simulink model "motor_kit_sim_20MHz"  (R2021b)
settings: Solver=VariableStepAuto  StartTime=0.0  StopTime=10*62.5E-6  RelTol=1e-3  EnableMultiTasking=on
PreLoadFcn:
  | setup_motor_kit_sim_20MHz;
InitFcn:
  | setup_motor_kit_sim_20MHz;
values from neighbouring files (symbols this model uses):
  DSPBASampleTime = 0.05e-6    (= 5e-08)    [setup_motor_kit_sim_20MHz.m]
  wordLength = 16    [setup_motor_kit_sim_20MHz.m]
undefined symbols (not defined in the file or in its folder): AdvDSPBChannelOutDisplay, dpoly, dspba_ChannelInVis, dspba_ChannelOutVis, dspba_internal_get_channel_ports, evalAionMaskParam, latency, primtype, value, x
libraries: DSPBAPrim x324, DSPBAModelBus x25, DSPBABase x7, dspsrcs4 x3, simulink x3, DSPBAUtilities x1
(part 1 of 5)
settings Model: Creator=ksmith  LastModifiedBy=alexhunt
settings SolverCC: AlgebraicLoopSolver=TrustRegion
settings DataIOCC: LimitDataPoints=on  SaveFormat=StructureWithTime  SignalLoggingSaveFormat=ModelDataLogs  ReturnWorkspaceOutputs=off
settings OptimizationCC: ExpressionDepthLimit=2147483647  LifeSpan=inf
settings DebuggingCC: UnderspecifiedInitializationDetection=Classic  MergeDetectMultiDrivingBlocksExec=none  SolverPrmCheckMsg=warning  FcnCallInpInsideContextMsg=warning  StateNameClashWarn=warning  SFUnexpectedBacktrackingDiag=warning  SFNoUnconditionalDefaultTransitionDiag=warning  SFExecutionAtInitializationDiag=none  SFMachineParentedDataDiag=warning  ArithmeticOperatorsInVariantConditions=warning
settings HardwareCC: ProdBitPerPointer=32  ProdBitPerSizeT=32  ProdBitPerPtrDiffT=32  ProdLargestAtomicFloat=None  ProdIntDivRoundTo=Undefined  ProdEndianess=Unspecified  ProdWordSize=32  ProdHWDeviceType=32-bit Generic
settings ModelReferenceCC: PropagateSignalLabelsOutOfModel=off
settings SFSimCC: SimUseLocalCustomCode=off  CustomCodeUndefinedFunction=UseInterfaceOnly
settings RTWCC: RTWUseLocalCustomCode=off
settings CodeAppCC: StateflowObjectComments=on
settings GRTTargetCC: TargetLangStandard=C89/C90 (ANSI)  CombineOutputUpdateFcns=off  GRTInterface=on
settings ConfigComp: CovMetricSettings=dw  CovSaveCumulativeToWorkspaceVar=on  CovSaveSingleToWorkspaceVar=on  CovExternalEMLEnable=off

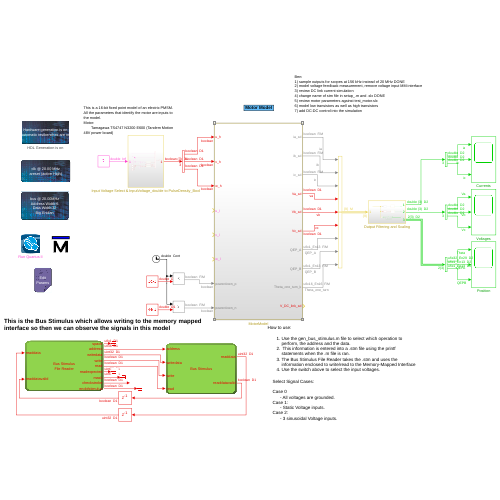
[thumbnail: Simulink's stored preview of the top-level diagram]
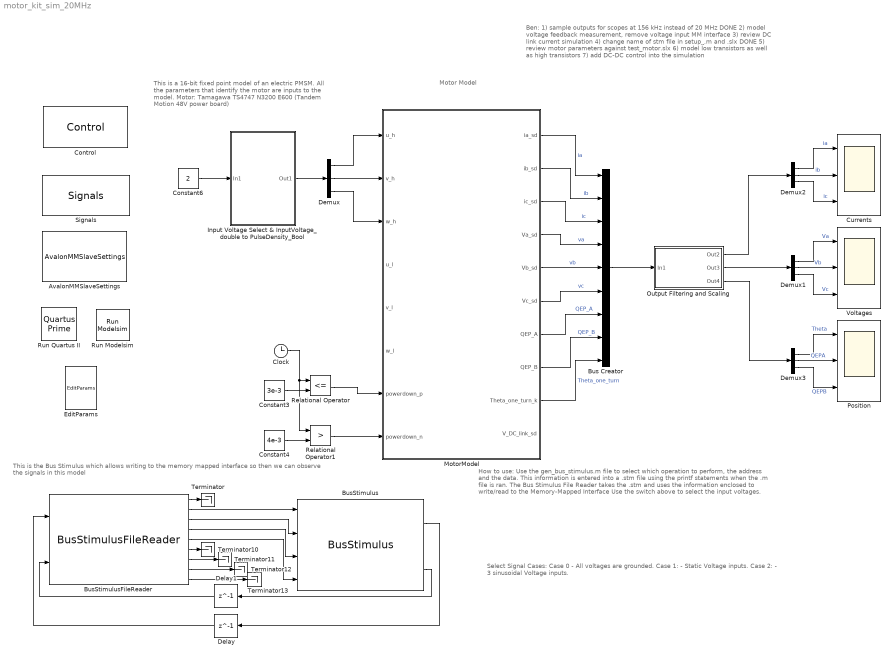
== system motor_kit_sim_20MHz ==
  note: Ben:
      | 1) sample outputs for scopes at 156 kHz instead of 20 MHz DONE
      | 2) model voltage feedback measurement, remove voltage input MM interface
      | 3) review DC link current simulation
      | 4) change name of stm file in setup_.m and .slx DONE
      | 5) review motor parameters against test_motor.slx
      | 6) model low transistors as well as high transistors
      | 7) add DC-DC control into the simulation
  note: How to use:
      |
      | Use the gen_bus_stimulus.m file to select which operation to perform, the address and the data.
      | This information is entered into a .stm file using the printf statements when the .m file is ran.
      | The Bus Stimulus File Reader takes the .stm and uses the information enclosed to write/read to the Memory-Mapped Interface
      | Use the switch above to select the input voltages.
  note: This is the Bus Stimulus which allows writing to the memory mapped interface so then we can observe the signals in this model
  note: This is a 16-bit fixed point model of an electric PMSM.
      | All the parameters that identify the motor are inputs to the model.
      | Motor:
      | 	Tamagawa TS4747 N3200 E600 (Tandem Motion 48V power board)
  note: Motor Model
  note: Select Signal Cases:
      |
      | Case 0
      | - All voltages are grounded.
      | Case 1:
      | - Static Voltage inputs.
      | Case 2:
      | - 3 sinusoidal Voltage inputs.
  AvalonMMSlaveSettings : DSPBABase/AvalonMMSlaveSettings
  Bus Creator : BusCreator  Inputs=9
  BusStimulus : DSPBAModelBus/BusStimulus  SampleTime=DSPBASampleTime  version=20140122  hasreaden=on
  BusStimulusFileReader : DSPBAModelBus/BusStimulusFileReader  enabled=on  filename=.\motor_kit_sim_20MHz_Autogen.stm  logfilename=.\test_bus_stimulus.bus.log  spacewidth=1  addrwidth=6  datawidth=32  SampleTime=DSPBASampleTime  version=20140124  hasreaden=on
  Clock : Clock
  Constant3 : Constant  Value=3e-3  OutDataTypeStr=double  SampleTime=DSPBASampleTime
  Constant4 : Constant  Value=4e-3  OutDataTypeStr=double  SampleTime=DSPBASampleTime
  Constant6 : Constant  Value=2
  Control : DSPBABase/Control  generate=on  language=VHDL  destination=./rtlmax10  destination_gui=./rtlmax10  make_full_path=off  path_is_relative=on  autotestbench=on  signaldepth=2  coveragetestbench=off  logs=off  spacewidth=2  spacenum=1  addrwidth=6  datawidth=32  dataendian=Big Endian  hierarchicalnames=off  ramThresholdBits=-1  distRamThresholdBits=-1  mlabThresholdBits=-1  hardMultiplierThresholdLuts=-1  version=20090407  errorOnChanMismatch=1  errorOnGPIOMismatch=0  importModelsimResults=0  cycleAccurate=off  reinterpretCastMult=off  paramFile=motor_kit_sim_20MHz_params.xml
      settings: AttributesFormatString=HDL Generation is %<generate>
  Currents : Scope  NumInputPorts=3
  Delay : Delay  DelayLength=1  InitialCondition=0
  Delay1 : Delay  DelayLength=1  InitialCondition=0
  Demux{,1..3} (4 alike) : Demux  Outputs=3
  EditParams : DSPBABase/EditParams  version=20090407
  Input Voltage Select & InputVoltage_double to PulseDensity_Bool : Subsystem
  MotorModel : Subsystem
  Output Filtering and Scaling : Subsystem
  Position : Scope  NumInputPorts=3
  Relational Operator : RelationalOperator  Operator=<=  OutDataTypeStr=boolean  RndMeth=Simplest
  Relational Operator1 : RelationalOperator  Operator=>  OutDataTypeStr=boolean  RndMeth=Simplest
  Run Modelsim : DSPBABase/Run Modelsim  version=20090407
  Run Quartus II : DSPBABase/Quartus Prime  version=20090407
  Signals : DSPBABase/Signals  clk=clk  freq=ClockFrequency  margin=0  rst=areset  rstactive=High  bus=bus  enbusclock=off  busfreq=20  bussync=on  version=20090407
  Terminator{,10..13} (5 alike) : Terminator
  Voltages : Scope  NumInputPorts=3
  wires:
  BusStimulusFileReader/2 -> BusStimulus/1
  BusStimulusFileReader/3 -> BusStimulus/2
  BusStimulusFileReader/4 -> BusStimulus/3
  BusStimulusFileReader/1 -> Terminator/1
  BusStimulusFileReader/6 -> Terminator10/1
  BusStimulusFileReader/7 -> Terminator11/1
  BusStimulusFileReader/8 -> Terminator12/1
  BusStimulusFileReader/9 -> Terminator13/1
  Delay/1 -> BusStimulusFileReader/1
  Delay1/1 -> BusStimulusFileReader/2
  BusStimulus/2 -> Delay1/1
  BusStimulus/1 -> Delay/1
  Demux/1 -> MotorModel/1(u_h)
  Demux/2 -> MotorModel/2(v_h)
  Demux/3 -> MotorModel/3(w_h)
  Demux1/1 -> Voltages/1  "Va"
  Demux1/2 -> Voltages/2  "Vb"
  Demux1/3 -> Voltages/3  "Vc"
  Demux2/1 -> Currents/1  "ia"
  Demux2/2 -> Currents/2  "ib"
  Demux2/3 -> Currents/3  "ic"
  Constant6/1 -> Input Voltage Select & InputVoltage_double to PulseDensity_Bool/1(In1)
  MotorModel/1(ia_sd) -> Bus Creator/1  "ia"
  MotorModel/2(ib_sd) -> Bus Creator/2  "ib"
  MotorModel/3(ic_sd) -> Bus Creator/3  "ic"
  MotorModel/4(Va_sd) -> Bus Creator/4  "va"
  MotorModel/5(Vb_sd) -> Bus Creator/5  "vb"
  MotorModel/6(Vc_sd) -> Bus Creator/6  "vc"
  MotorModel/7(QEP_A) -> Bus Creator/7  "QEP_A"
  MotorModel/8(QEP_B) -> Bus Creator/8  "QEP_B"
  MotorModel/9(Theta_one_turn_k) -> Bus Creator/9  "Theta_one_turn"
  Bus Creator/1 -> Output Filtering and Scaling/1(In1)
  Demux3/1 -> Position/1  "Theta"
  Demux3/2 -> Position/2  "QEPA"
  Demux3/3 -> Position/3  "QEPB"
  Output Filtering and Scaling/1(Out2) -> Demux2/1
  Output Filtering and Scaling/2(Out3) -> Demux1/1
  Output Filtering and Scaling/3(Out4) -> Demux3/1
  Input Voltage Select & InputVoltage_double to PulseDensity_Bool/1(Out1) -> Demux/1
  BusStimulusFileReader/5 -> BusStimulus/4
  Clock/1 -> Relational Operator1/1, Relational Operator/1
  Constant3/1 -> Relational Operator/2
  Constant4/1 -> Relational Operator1/2
  Relational Operator/1 -> MotorModel/7(powerdown_p)
  Relational Operator1/1 -> MotorModel/8(powerdown_n)

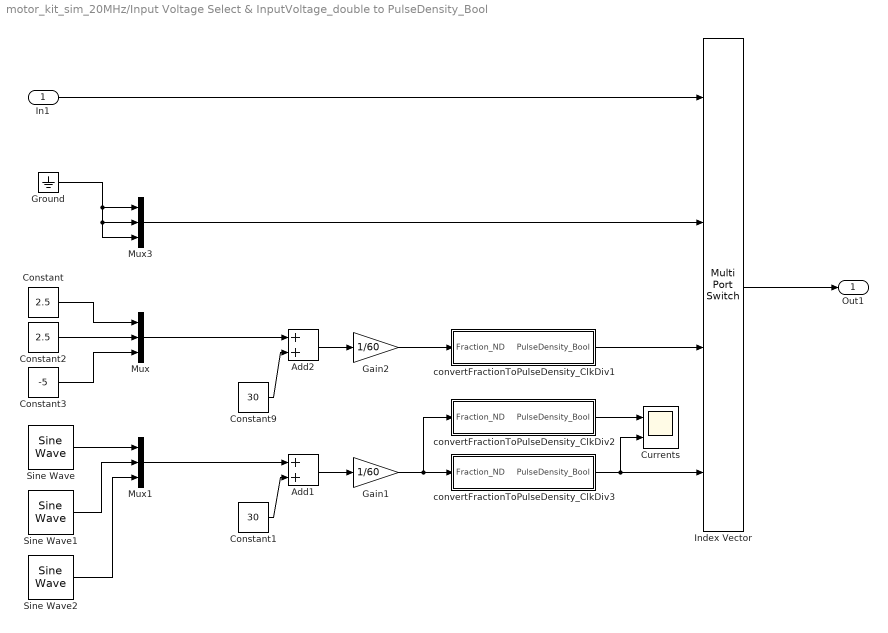
== system motor_kit_sim_20MHz/Input Voltage Select & InputVoltage_double to PulseDensity_Bool ==
  In1 : Inport
  Add1 : Sum
  Add2 : Sum
  Constant : Constant  Value=2.5
  Constant1 : Constant  Value=30
  Constant2 : Constant  Value=2.5
  Constant3 : Constant  Value=-5
  Constant9 : Constant  Value=30
  Currents : Scope  NumInputPorts=2
  Gain1 : Gain  Gain=1/60
  Gain2 : Gain  Gain=1/60
  Ground : Ground
  Index Vector : MultiPortSwitch  DataPortOrder=Zero-based contiguous  zeroidx=on
  Mux : Mux  Inputs=3
  Mux1 : Mux  Inputs=3
  Mux3 : Mux  Inputs=3
  Sine Wave : dspsrcs4/Sine Wave  Amplitude=2  Frequency=16.6  Phase=0  SampleMode=Discrete  OutComplex=Real  CompMethod=Trigonometric fcn  TableSize=Speed  SampleTime=1/20000000  SamplesPerFrame=1  ResetState=Restart at time zero  OutputFrames=off  dataType=double  wordLen=16  udDataType=sfix(16)  fracBitsMode=Best precision  numFracBits=15  OutDataTypeStr=double  LastOutDataTypeStr=double
  Sine Wave1 : dspsrcs4/Sine Wave  Amplitude=2  Frequency=16.6  Phase=2.094  SampleMode=Discrete  OutComplex=Real  CompMethod=Trigonometric fcn  TableSize=Speed  SampleTime=1/20000000  SamplesPerFrame=1  ResetState=Restart at time zero  OutputFrames=off  dataType=double  wordLen=16  udDataType=sfix(16)  fracBitsMode=Best precision  numFracBits=15  OutDataTypeStr=double  LastOutDataTypeStr=double
  Sine Wave2 : dspsrcs4/Sine Wave  Amplitude=2  Frequency=16.6  Phase=4.189  SampleMode=Discrete  OutComplex=Real  CompMethod=Trigonometric fcn  TableSize=Speed  SampleTime=1/20000000  SamplesPerFrame=1  ResetState=Restart at time zero  OutputFrames=off  dataType=double  wordLen=16  udDataType=sfix(16)  fracBitsMode=Best precision  numFracBits=15  OutDataTypeStr=double  LastOutDataTypeStr=double
  convertFractionToPulseDensity_ClkDiv1 : Subsystem
  convertFractionToPulseDensity_ClkDiv2 : Subsystem
  convertFractionToPulseDensity_ClkDiv3 : Subsystem
  Out1 : Outport
  wires:
  Add2/1 -> Gain2/1
  Constant9/1 -> Add2/2
  Gain2/1 -> convertFractionToPulseDensity_ClkDiv1/1(Fraction_ND)
  Constant1/1 -> Add1/2
  Add1/1 -> Gain1/1
  Mux1/1 -> Add1/1
  Constant2/1 -> Mux/2
  Constant/1 -> Mux/1
  Mux/1 -> Add2/1
  Constant3/1 -> Mux/3
  Sine Wave/1 -> Mux1/1
  Sine Wave1/1 -> Mux1/2
  Sine Wave2/1 -> Mux1/3
  convertFractionToPulseDensity_ClkDiv1/1(PulseDensity_Bool) -> Index Vector/3
  In1/1 -> Index Vector/1
  Ground/1 -> Mux3/3, Mux3/2, Mux3/1
  Mux3/1 -> Index Vector/2
  Index Vector/1 -> Out1/1
  convertFractionToPulseDensity_ClkDiv3/1(PulseDensity_Bool) -> Currents/2, Index Vector/4
  Gain1/1 -> convertFractionToPulseDensity_ClkDiv2/1(Fraction_ND), convertFractionToPulseDensity_ClkDiv3/1(Fraction_ND)
  convertFractionToPulseDensity_ClkDiv2/1(PulseDensity_Bool) -> Currents/1

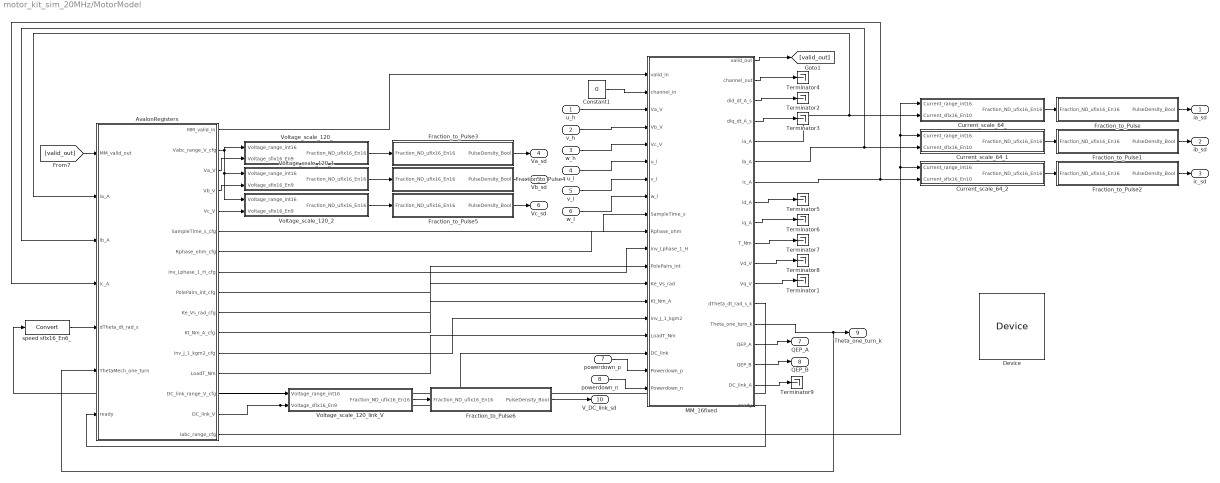
== system motor_kit_sim_20MHz/MotorModel ==
  u_h : Inport  OutDataTypeStr=boolean
  v_h : Inport  Port=2  OutDataTypeStr=boolean
  w_h : Inport  Port=3  OutDataTypeStr=boolean
  u_l : Inport  Port=4  OutDataTypeStr=boolean  PortDimensions=1
  v_l : Inport  Port=5  OutDataTypeStr=boolean  PortDimensions=1
  w_l : Inport  Port=6  OutDataTypeStr=boolean  PortDimensions=1
  powerdown_p : Inport  Port=7  OutDataTypeStr=boolean  PortDimensions=1
  powerdown_n : Inport  Port=8  OutDataTypeStr=boolean  PortDimensions=1
  AvalonRegisters : Subsystem
  Constant1 : Constant  Value=0  OutDataTypeStr=uint8
  Current_scale_64_ : Subsystem
  Current_scale_64_1 : Subsystem
  Current_scale_64_2 : Subsystem
  Device : DSPBABase/Device  family=MAX 10  deviceMember=Stratix V GX  stratix4device=Stratix IV E  hardcopy4device=HardCopy IV E  stratix5device=Stratix V GX  device=AUTO  speed=6  stratixSpeed=-5  stratix2Speed=-3  stratix3Speed=-2  stratix4gxSpeed=-2  stratix4gtSpeed=-1  cyclone2Speed=-6  cyclone3Speed=-7  arria2Speed=-4  cyclone4eSpeed=-8  stratix5Speed=-3  arria5Speed=-4  arriaSpeed=-6  cyclone3lsSpeed=-7  cyclone5Speed=-6  arria2gzSpeed=-3  nightFurySpeed=-2  ecp2Speed=-7  hardcopycompat=off  version=20140217  max10flashmode=off  max10nomeminit=off
  Fraction_to_Pulse : Subsystem
  Fraction_to_Pulse1 : Subsystem
  Fraction_to_Pulse2 : Subsystem
  Fraction_to_Pulse3 : Subsystem
  Fraction_to_Pulse4 : Subsystem
  Fraction_to_Pulse5 : Subsystem
  Fraction_to_Pulse6 : Subsystem
  MM_16fixed : Subsystem
  Terminator{1..9} (9 alike) : Terminator
  Voltage_scale_120_ : Subsystem
  Voltage_scale_120_1 : Subsystem
  Voltage_scale_120_2 : Subsystem
  Voltage_scale_120_link_V : Subsystem
  speed sfix16_En6_ : DSPBAPrim/Convert  primtype=convert  nInputs=1  nOutputs=1  omode=Specify via dialog  otype=sfix(16)  scale=2^-6  rndmethod=Unbiased  factor=1  satmethod=None  shift_vec=[0 1 2 -1]  value=round([0:255]/17)  inPortNames=[' '; ' ';]  outPortNames=[' '; 'c']  dspbaimage=dspba_prim_wide.svg  text=fprintf('convert');  style=Optimised  visibilities=8+64+256+2^17  clipdetect=off  floatPrecision=float32_m23  advOptions=[]  version=20211007
  ia_sd : Outport
  ib_sd : Outport  Port=2
  ic_sd : Outport  Port=3
  Va_sd : Outport  Port=4
  Vb_sd : Outport  Port=5
  Vc_sd : Outport  Port=6
  QEP_A : Outport  Port=7
  QEP_B : Outport  Port=8
  Theta_one_turn_k : Outport  Port=9
  V_DC_link_sd : Outport  Port=10
  wires:
  Fraction_to_Pulse4/1("PulseDensity_Bool ") -> Vb_sd/1
  Fraction_to_Pulse2/1("PulseDensity_Bool ") -> ic_sd/1
  MM_16fixed/6(ib_A) -> AvalonRegisters/3(ib_A), Current_scale_64_1/2(Current_sfix16_En10)
  MM_16fixed/7(ic_A) -> Current_scale_64_2/2(Current_sfix16_En10), AvalonRegisters/4(ic_A)
  MM_16fixed/12(Vq_V) -> Terminator1/1
  [valid_out] -> AvalonRegisters/1(MM_valid_out)
  MM_16fixed/9(iq_A) -> Terminator6/1
  MM_16fixed/13(dTheta_dt_rad_s_k) -> speed sfix16_En6_/1
  MM_16fixed/4(diq_dt_A_s) -> Terminator3/1
  MM_16fixed/3(did_dt_A_s) -> Terminator2/1
  MM_16fixed/10(T_Nm) -> Terminator7/1
  AvalonRegisters/9(PolePairs_int_cfg) -> MM_16fixed/12(PolePairs_int)
  AvalonRegisters/12(inv_J_1_kgm2_cfg) -> MM_16fixed/15(inv_J_1_kgm2)
  AvalonRegisters/1(MM_valid_in) -> MM_16fixed/1(valid_in)
  AvalonRegisters/10(Ke_Vs_rad_cfg) -> MM_16fixed/13(Ke_Vs_rad)
  AvalonRegisters/8(inv_Lphase_1_H_cfg) -> MM_16fixed/11(inv_Lphase_1_H)
  Fraction_to_Pulse5/1("PulseDensity_Bool ") -> Vc_sd/1
  AvalonRegisters/11(Kt_Nm_A_cfg) -> MM_16fixed/14(Kt_Nm_A)
  AvalonRegisters/7(Rphase_ohm_cfg) -> MM_16fixed/10(Rphase_ohm)
  Fraction_to_Pulse1/1("PulseDensity_Bool ") -> ib_sd/1
  MM_16fixed/5(ia_A) -> Current_scale_64_/2(Current_sfix16_En10), AvalonRegisters/2(ia_A)
  MM_16fixed/11(Vd_V) -> Terminator8/1
  MM_16fixed/2(channel_out) -> Terminator4/1
  AvalonRegisters/6(SampleTime_s_cfg) -> MM_16fixed/9(SampleTime_s)
  speed sfix16_En6_/1 -> AvalonRegisters/5(dTheta_dt_rad_s)
  MM_16fixed/8(id_A) -> Terminator5/1
  AvalonRegisters/13(LoadT_Nm) -> MM_16fixed/16(LoadT_Nm)
  MM_16fixed/18(ready) -> AvalonRegisters/7(ready)
  MM_16fixed/1(valid_out) -> [valid_out]
  Constant1/1 -> MM_16fixed/2(channel_in)
  MM_16fixed/15(QEP_A) -> QEP_A/1
  MM_16fixed/16(QEP_B) -> QEP_B/1
  MM_16fixed/14(Theta_one_turn_k) -> AvalonRegisters/6(ThetaMech_one_turn), Theta_one_turn_k/1
  v_h/1 -> MM_16fixed/4(Vb_V)
  w_h/1 -> MM_16fixed/5(Vc_V)
  Fraction_to_Pulse3/1("PulseDensity_Bool ") -> Va_sd/1
  Fraction_to_Pulse/1("PulseDensity_Bool ") -> ia_sd/1
  u_h/1 -> MM_16fixed/3(Va_V)
  Voltage_scale_120_/1("Fraction_ND_ufix16_En16 ") -> Fraction_to_Pulse3/1(Fraction_ND_ufix16_En16)
  Voltage_scale_120_2/1("Fraction_ND_ufix16_En16 ") -> Fraction_to_Pulse5/1(Fraction_ND_ufix16_En16)
  Voltage_scale_120_1/1("Fraction_ND_ufix16_En16 ") -> Fraction_to_Pulse4/1(Fraction_ND_ufix16_En16)
  Current_scale_64_1/1("Fraction_ND_ufix16_En16 ") -> Fraction_to_Pulse1/1(Fraction_ND_ufix16_En16)
  Current_scale_64_/1("Fraction_ND_ufix16_En16 ") -> Fraction_to_Pulse/1(Fraction_ND_ufix16_En16)
  Current_scale_64_2/1("Fraction_ND_ufix16_En16 ") -> Fraction_to_Pulse2/1(Fraction_ND_ufix16_En16)
  AvalonRegisters/15(DC_link_V) -> MM_16fixed/17(DC_link), Voltage_scale_120_link_V/2(Voltage_sfix16_En9)
  w_l/1 -> MM_16fixed/8(w_l)
  v_l/1 -> MM_16fixed/7(v_l)
  u_l/1 -> MM_16fixed/6(u_l)
  Voltage_scale_120_link_V/1("Fraction_ND_ufix16_En16 ") -> Fraction_to_Pulse6/1(Fraction_ND_ufix16_En16)
  Fraction_to_Pulse6/1("PulseDensity_Bool ") -> V_DC_link_sd/1
  MM_16fixed/17(DC_link_A) -> Terminator9/1
  AvalonRegisters/5(Vc_V) -> Voltage_scale_120_2/2(Voltage_sfix16_En9)
  AvalonRegisters/4(Vb_V) -> Voltage_scale_120_1/2(Voltage_sfix16_En9)
  AvalonRegisters/3(Va_V) -> Voltage_scale_120_/2(Voltage_sfix16_En9)
  AvalonRegisters/2(Vabc_range_V_cfg) -> Voltage_scale_120_2/1(Voltage_range_int16), Voltage_scale_120_1/1(Voltage_range_int16), Voltage_scale_120_/1(Voltage_range_int16)
  AvalonRegisters/14(DC_link_range_V_cfg) -> Voltage_scale_120_link_V/1(Voltage_range_int16)
  AvalonRegisters/16(Iabc_range_cfg) -> Current_scale_64_/1(Current_range_int16), Current_scale_64_1/1(Current_range_int16), Current_scale_64_2/1(Current_range_int16)
  powerdown_p/1 -> MM_16fixed/18(Powerdown_p)
  powerdown_n/1 -> MM_16fixed/19(Powerdown_n)

== system motor_kit_sim_20MHz/Output Filtering and Scaling ==
  In1 : Inport
  Bus Creator : BusCreator  Inputs=3
  Bus Selector : BusSelector  OutputSignals=ia,ib,ic  OutputAsBus=on
  Bus Selector1 : BusSelector  OutputSignals=va,vb,vc  OutputAsBus=on
  Bus Selector2 : BusSelector  OutputSignals=Theta_one_turn,QEP_A,QEP_B
  Data Type Conversion : DataTypeConversion  OutDataTypeStr=double
  Data Type Conversion1 : DataTypeConversion  OutDataTypeStr=double
  Gain3 : Gain  Gain=2*pi
  Sinc3 Filter : Subsystem
  Sinc3 Filter1 : Subsystem
  Zero-Order Hold : ZeroOrderHold  SampleTime=128*DSPBASampleTime
  Out2 : Outport
  Out3 : Outport  Port=2
  Out4 : Outport  Port=3
  wires:
  Bus Selector/1 -> Data Type Conversion/1
  Bus Selector1/1 -> Data Type Conversion1/1
  Bus Selector2/1 -> Gain3/1  "<Theta_one_turn>"
  Gain3/1 -> Bus Creator/1
  Bus Selector2/3 -> Bus Creator/3  "<QEP_B>"
  Bus Selector2/2 -> Bus Creator/2  "<QEP_A>"
  Bus Creator/1 -> Out4/1
  In1/1 -> Zero-Order Hold/1, Bus Selector1/1, Bus Selector/1
  Data Type Conversion1/1 -> Sinc3 Filter/1(In1)
  Data Type Conversion/1 -> Sinc3 Filter1/1(In1)
  Sinc3 Filter1/1(Out1) -> Out2/1
  Sinc3 Filter/1(Out1) -> Out3/1
  Zero-Order Hold/1 -> Bus Selector2/1

== system motor_kit_sim_20MHz/Input Voltage Select & InputVoltage_double to PulseDensity_Bool/convertFractionToPulseDensity_ClkDiv1 ==
  note: Subtract threshold once it is reached
  note: Each timestep:
      | Calculate the new value of the integral:
      | New value (temp) =  Old value + input*timestep
      | If the new value exceeds the threshold:
      | 1. Set output to 1
      | 2. Decrease the integral by the threshold:
      | New value (final) =  New value (temp) - threshold
      | Else
      | 1. Set output to zero
      | 2. New value (final) =  New value (temp)
  Fraction_ND : Inport
  Compare To Threshold : simulink/Logic and Bit Operations/Compare To Constant  relop=>=  const=1  OutDataTypeStr=boolean
  Constant : Constant
  Constant1 : Constant  Value=0
  Rate Transition : RateTransition  OutPortSampleTime=DSPBASampleTime
  Rate Transition1 : RateTransition  OutPortSampleTime=DSPBASampleTime
  Sum : Sum  Inputs=+-
  Sum1 : Sum
  Switch : Switch  Criteria=u2 > Threshold
  Unit Delay1 : UnitDelay  SampleTime=-1  HasFrameUpgradeWarning=on
  PulseDensity_Bool : Outport
  wires:
  Switch/1 -> Sum/2
  Constant1/1 -> Switch/3
  Constant/1 -> Switch/1
  Unit Delay1/1 -> Sum1/2, Compare To Threshold/1
  Sum1/1 -> Unit Delay1/1
  Compare To Threshold/1 -> Switch/2, Rate Transition/1
  Fraction_ND/1 -> Rate Transition1/1
  Sum/1 -> Sum1/1
  Rate Transition1/1 -> Sum/1
  Rate Transition/1 -> PulseDensity_Bool/1

== system motor_kit_sim_20MHz/Input Voltage Select & InputVoltage_double to PulseDensity_Bool/convertFractionToPulseDensity_ClkDiv2 ==
  note: Subtract threshold once it is reached
  note: Each timestep:
      | Calculate the new value of the integral:
      | New value (temp) =  Old value + input*timestep
      | If the new value exceeds the threshold:
      | 1. Set output to 1
      | 2. Decrease the integral by the threshold:
      | New value (final) =  New value (temp) - threshold
      | Else
      | 1. Set output to zero
      | 2. New value (final) =  New value (temp)
  Fraction_ND : Inport
  Compare To Threshold : simulink/Logic and Bit Operations/Compare To Constant  relop=>=  const=1  OutDataTypeStr=boolean
  Constant : Constant
  Constant1 : Constant  Value=0
  Rate Transition : RateTransition  OutPortSampleTime=DSPBASampleTime
  Rate Transition1 : RateTransition  OutPortSampleTime=DSPBASampleTime
  Sum : Sum  Inputs=+-
  Sum1 : Sum
  Switch : Switch  Criteria=u2 > Threshold
  Unit Delay1 : UnitDelay  SampleTime=-1  HasFrameUpgradeWarning=on
  PulseDensity_Bool : Outport
  wires:
  Rate Transition/1 -> PulseDensity_Bool/1
  Switch/1 -> Sum/2
  Constant1/1 -> Switch/3
  Constant/1 -> Switch/1
  Unit Delay1/1 -> Sum1/2, Compare To Threshold/1
  Sum1/1 -> Unit Delay1/1
  Compare To Threshold/1 -> Switch/2, Rate Transition/1
  Fraction_ND/1 -> Rate Transition1/1
  Sum/1 -> Sum1/1
  Rate Transition1/1 -> Sum/1

== system motor_kit_sim_20MHz/Input Voltage Select & InputVoltage_double to PulseDensity_Bool/convertFractionToPulseDensity_ClkDiv3 ==
  note: Subtract threshold once it is reached
  note: Each timestep:
      | Calculate the new value of the integral:
      | New value (temp) =  Old value + input*timestep
      | If the new value exceeds the threshold:
      | 1. Set output to 1
      | 2. Decrease the integral by the threshold:
      | New value (final) =  New value (temp) - threshold
      | Else
      | 1. Set output to zero
      | 2. New value (final) =  New value (temp)
  Fraction_ND : Inport
  Rate Transition : RateTransition  OutPortSampleTime=DSPBASampleTime
  Rate Transition1 : RateTransition  OutPortSampleTime=DSPBASampleTime
  Relational Operator2 : RelationalOperator  Operator=>  OutDataTypeStr=boolean  RndMeth=Nearest
  Vtri2 : simulink/Sources/Repeating Sequence  rep_seq_t=[0 1/16000 1/8000 ]  rep_seq_y=[0 1 0]
  PulseDensity_Bool : Outport
  wires:
  Rate Transition/1 -> PulseDensity_Bool/1
  Relational Operator2/1 -> Rate Transition/1
  Fraction_ND/1 -> Rate Transition1/1
  Rate Transition1/1 -> Relational Operator2/1
  Vtri2/1 -> Relational Operator2/2

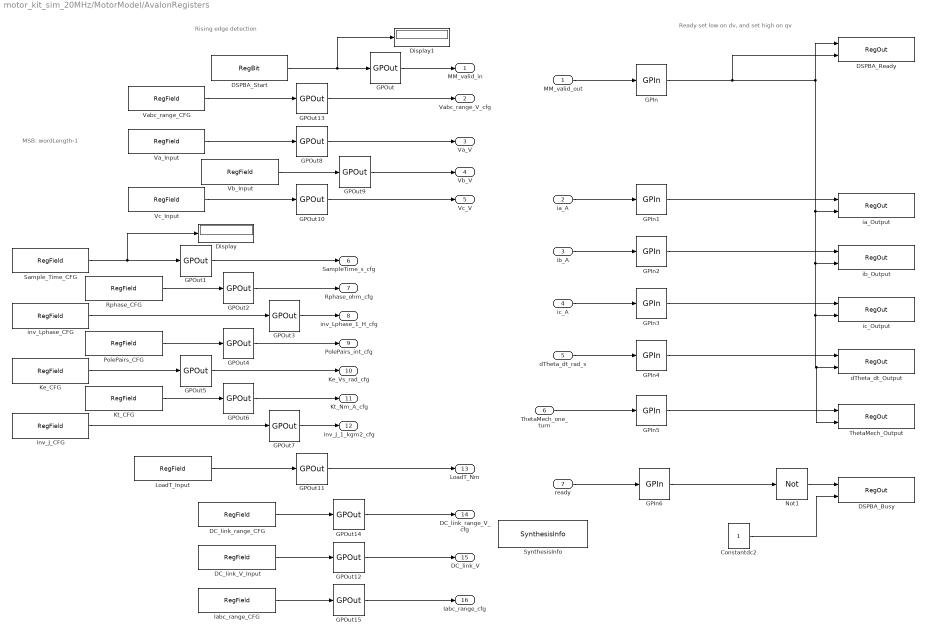
== system motor_kit_sim_20MHz/MotorModel/AvalonRegisters ==
  note: MSB: wordLength-1
  note: Rising edge detection
  note: Ready set low on dv, and set high on qv
  MM_valid_out : Inport
  ia_A : Inport  Port=2
  ib_A : Inport  Port=3
  ic_A : Inport  Port=4
  dTheta_dt_rad_s : Inport  Port=5
  ThetaMech_one_turn : Inport  Port=6
  ready : Inport  Port=7
  Constantdc2 : Constant  OutDataTypeStr=boolean  SampleTime=DSPBASampleTime
  DC_link_V_Input : DSPBAModelBus/RegField  reg_name=DC_link_V  reg_rwmode=Read/Write  reg_msb=wordLength - 1  reg_lsb=0  reg_mode=Specify via dialog  reg_type=DataType  reg_scale=constScaleVoltage  reg_init=0  reg_desc=DC link input value  reg_modal=off  reg_desc0=0  reg_desc1=0  reg_desc2=0  reg_desc3=0  reg_desc4=0  reg_desc5=0  reg_desc6=0  reg_desc7=0  reg_addr=37  SampleTime=DSPBASampleTime  version=20090407
  DC_link_range_CFG : DSPBAModelBus/RegField  reg_name=DC_link_range_cfg  reg_rwmode=Read/Write  reg_msb=wordLength - 1  reg_lsb=0  reg_mode=Specify via dialog  reg_type=DataType  reg_scale=constScaleVoltage_range  reg_init=0  reg_desc=DC link range input value  reg_modal=off  reg_desc0=0  reg_desc1=0  reg_desc2=0  reg_desc3=0  reg_desc4=0  reg_desc5=0  reg_desc6=0  reg_desc7=0  reg_addr=38  SampleTime=DSPBASampleTime  version=20090407
  DSPBA_Busy : DSPBAModelBus/RegOut  reg_name=Busy  reg_rwmode=Read  reg_msb=0  reg_lsb=0  reg_desc=Busy bit - When '1' not ready to accept new data  reg_addr=0  SampleTime=-1  version=20090407
  DSPBA_Ready : DSPBAModelBus/RegOut  reg_name=Ready  reg_rwmode=Read  reg_msb=0  reg_lsb=0  reg_desc=Ready bit - Output data is ready when 'Control' reg value matches 'Ready'  reg_addr=3  SampleTime=-1  version=20090407
  DSPBA_Start : DSPBAModelBus/RegBit  reg_name=Start  reg_rwmode=Read/Write  reg_lsb=0  reg_init=0  reg_desc=Start bit - toggle bit value once to start  reg_addr=1  reg_desc0=0  reg_desc1=0  SampleTime=DSPBASampleTime  version=20090407
  Display : Display
  Display1 : Display
  GPIn{,1..6} (7 alike) : DSPBAPrim/GPIn  primtype=gpin  nInputs=evalAionMaskParam(gcb,'value',1)  nOutputs=evalAionMaskParam(gcb,'value',1)  omode=Inherit via internal rule  otype=sfix(16)  scale=2^-15  rndmethod=Unbiased  factor=1  satmethod=Symmetric  shift_vec=[0 1 2 -1]  value=1  inPortNames=[' ' ' ' ' ' ' ' ' ' ' ' ' ' ' ' ' ' ' ' ' ' ' ' ' ' ' ' ' ' ' ' ' ' ' ' ' ' ' ' ' ' ' ' ' ' ' ' ' ' ' ' ' ' ' ' ' ' ' ' ' ' ' ' ' ' ' ' ' ']'  outPortNames=[' ' ' ' ' ' ' ' ' ' ' ' ' ' ' ' ' ' ' ' ' ' ' ' ' ' ' ' ' ' ' ' ' ' ' ' ' ' ' ' ' ' ' ' ' ' ' ' ' ' ' ' ' ' ' ' ' ' ' ' ' ' ' ' ' ' ' ' ' ']'  dspbaimage=dspba_prim_channel_tall.svg  text=fprintf('GPIn');  style=Optimised  visibilities=1024  scheduleOrigin=off  version=20211214
  GPOut{,1..15} (16 alike) : DSPBAPrim/GPOut  primtype=gpout  nInputs=evalAionMaskParam(gcb,'value',1)  nOutputs=evalAionMaskParam(gcb,'value',1)  omode=Inherit via internal rule  otype=sfix(16)  scale=2^-15  rndmethod=Unbiased  factor=1  satmethod=Symmetric  shift_vec=[0 1 2 -1]  value=1  inPortNames=[' ' ' ' ' ' ' ' ' ' ' ' ' ' ' ' ' ' ' ' ' ' ' ' ' ' ' ' ' ' ' ' ' ' ' ' ' ' ' ' ' ' ' ' ' ' ' ' ' ' ' ' ' ' ' ' ' ' ' ' ' ' ' ' ' ' ' ' ' ']'  outPortNames=[' ' ' ' ' ' ' ' ' ' ' ' ' ' ' ' ' ' ' ' ' ' ' ' ' ' ' ' ' ' ' ' ' ' ' ' ' ' ' ' ' ' ' ' ' ' ' ' ' ' ' ' ' ' ' ' ' ' ' ' ' ' ' ' ' ' ' ' ' ']'  dspbaimage=dspba_prim_channel_tall.svg  text=fprintf('GPOut');  style=Optimised  visibilities=1024  latency=0  version=20211214
  Iabc_range_CFG : DSPBAModelBus/RegField  reg_name=Iabc_range_cfg  reg_rwmode=Read/Write  reg_msb=wordLength - 1  reg_lsb=0  reg_mode=Specify via dialog  reg_type=DataType  reg_scale=constScaleCurrent_range  reg_init=0  reg_desc=Iabc range input value  reg_modal=off  reg_desc0=0  reg_desc1=0  reg_desc2=0  reg_desc3=0  reg_desc4=0  reg_desc5=0  reg_desc6=0  reg_desc7=0  reg_addr=47  SampleTime=DSPBASampleTime  version=20090407
  Ke_CFG : DSPBAModelBus/RegField  reg_name=Ke_cfg  reg_rwmode=Read/Write  reg_msb=wordLength - 1  reg_lsb=0  reg_mode=Specify via dialog  reg_type=ufix(16)  reg_scale=2^-16  reg_init=0  reg_desc=Ke_cfg input value  reg_modal=off  reg_desc0=0  reg_desc1=0  reg_desc2=0  reg_desc3=0  reg_desc4=0  reg_desc5=0  reg_desc6=0  reg_desc7=0  reg_addr=20  SampleTime=DSPBASampleTime  version=20090407
  Kt_CFG : DSPBAModelBus/RegField  reg_name=Kt_cfg  reg_rwmode=Read/Write  reg_msb=wordLength - 1  reg_lsb=0  reg_mode=Specify via dialog  reg_type=ufix(16)  reg_scale=2^-16  reg_init=0  reg_desc=Kt_cfg input value  reg_modal=off  reg_desc0=0  reg_desc1=0  reg_desc2=0  reg_desc3=0  reg_desc4=0  reg_desc5=0  reg_desc6=0  reg_desc7=0  reg_addr=21  SampleTime=DSPBASampleTime  version=20090407
  LoadT_Input : DSPBAModelBus/RegField  reg_name=LoadT  reg_rwmode=Read/Write  reg_msb=wordLength - 1  reg_lsb=0  reg_mode=Specify via dialog  reg_type=DataType  reg_scale=constScaleTorque  reg_init=0  reg_desc=LoadT input value  reg_modal=off  reg_desc0=0  reg_desc1=0  reg_desc2=0  reg_desc3=0  reg_desc4=0  reg_desc5=0  reg_desc6=0  reg_desc7=0  reg_addr=35  SampleTime=DSPBASampleTime  version=20090407
  Not1 : DSPBAPrim/Not  primtype=not  nInputs=1  nOutputs=1  omode=Inherit via internal rule  otype=sfix(16)  scale=2^-15  rndmethod=Unbiased  factor=1  satmethod=Symmetric  shift_vec=[0 1 2 -1]  value=0  inPortNames=[' '; ' ';]  outPortNames=[' ']  dspbaimage=dspba_prim.svg  text=fprintf('~');  style=Optimised  visibilities=8  version=20211007
  PolePairs_CFG : DSPBAModelBus/RegField  reg_name=PolePairs_cfg  reg_rwmode=Read/Write  reg_msb=wordLength - 1  reg_lsb=0  reg_mode=Specify via dialog  reg_type=ufix(16)  reg_scale=2^-14  reg_init=0  reg_desc=PolePairs_cfg input value  reg_modal=off  reg_desc0=0  reg_desc1=0  reg_desc2=0  reg_desc3=0  reg_desc4=0  reg_desc5=0  reg_desc6=0  reg_desc7=0  reg_addr=19  SampleTime=DSPBASampleTime  version=20090407
  Rphase_CFG : DSPBAModelBus/RegField  reg_name=Rphase_cfg  reg_rwmode=Read/Write  reg_msb=wordLength - 1  reg_lsb=0  reg_mode=Specify via dialog  reg_type=ufix(16)  reg_scale=2^-16  reg_init=0  reg_desc=Rphase_cfg input value  reg_modal=off  reg_desc0=0  reg_desc1=0  reg_desc2=0  reg_desc3=0  reg_desc4=0  reg_desc5=0  reg_desc6=0  reg_desc7=0  reg_addr=17  SampleTime=DSPBASampleTime  version=20090407
  Sample_Time_CFG : DSPBAModelBus/RegField  reg_name=SampleTime_cfg  reg_rwmode=Read/Write  reg_msb=wordLength - 1  reg_lsb=0  reg_mode=Specify via dialog  reg_type=ufix(16)  reg_scale=2^-39  reg_init=0  reg_desc=SampleTime_cfg input value  reg_modal=off  reg_desc0=0  reg_desc1=0  reg_desc2=0  reg_desc3=0  reg_desc4=0  reg_desc5=0  reg_desc6=0  reg_desc7=0  reg_addr=16  SampleTime=DSPBASampleTime  version=20090407
  SynthesisInfo : DSPBAPrim/SynthesisInfo  primtype=synthinfo  nInputs=0  nOutputs=0  omode=Inherit via internal rule  otype=sfix(16)  scale=2^-15  rndmethod=Truncate  factor=1  satmethod=Symmetric  shift_vec=[0 1 2 -1]  value=99  inPortNames=[' '; ' ';]  outPortNames=[' ']  dspbaimage=dspba_prim_ctrl.jpg  text=fprintf('Style=%s', style);  style=Scheduled  visibilities=32768  constraintPair=None  constraintRelation=>  constraintLimit=2  modelRefSign=+  modelRef=''  showSchedule=off  simulationMode=Use Global Value  resetMinimization=Conditional - On for ChannelIn/Out only  version=20220106
  ThetaMech_Output : DSPBAModelBus/RegOut  reg_name=ThetaMech  reg_rwmode=Read  reg_msb=wordLength - 1  reg_lsb=0  reg_desc=ThetaMech one turn output value  reg_addr=55  SampleTime=-1  version=20090407
  Va_Input : DSPBAModelBus/RegField  reg_name=Va  reg_rwmode=Read/Write  reg_msb=wordLength - 1  reg_lsb=0  reg_mode=Specify via dialog  reg_type=DataType  reg_scale=constScaleVoltage  reg_init=0  reg_desc=Va input value  reg_modal=off  reg_desc0=0  reg_desc1=0  reg_desc2=0  reg_desc3=0  reg_desc4=0  reg_desc5=0  reg_desc6=0  reg_desc7=0  reg_addr=32  SampleTime=DSPBASampleTime  version=20090407
  Vabc_range_CFG : DSPBAModelBus/RegField  reg_name=Vabc_range_cfg  reg_rwmode=Read/Write  reg_msb=wordLength - 1  reg_lsb=0  reg_mode=Specify via dialog  reg_type=DataType  reg_scale=constScaleVoltage_range  reg_init=0  reg_desc=Vabc range Input value.  reg_modal=off  reg_desc0=0  reg_desc1=0  reg_desc2=0  reg_desc3=0  reg_desc4=0  reg_desc5=0  reg_desc6=0  reg_desc7=0  reg_addr=31  SampleTime=DSPBASampleTime  version=20090407
  Vb_Input : DSPBAModelBus/RegField  reg_name=Vb  reg_rwmode=Read/Write  reg_msb=wordLength - 1  reg_lsb=0  reg_mode=Specify via dialog  reg_type=DataType  reg_scale=constScaleVoltage  reg_init=0  reg_desc=Vb input value  reg_modal=off  reg_desc0=0  reg_desc1=0  reg_desc2=0  reg_desc3=0  reg_desc4=0  reg_desc5=0  reg_desc6=0  reg_desc7=0  reg_addr=33  SampleTime=DSPBASampleTime  version=20090407
  Vc_Input : DSPBAModelBus/RegField  reg_name=Vc  reg_rwmode=Read/Write  reg_msb=wordLength - 1  reg_lsb=0  reg_mode=Specify via dialog  reg_type=DataType  reg_scale=constScaleVoltage  reg_init=0  reg_desc=Vc input value  reg_modal=off  reg_desc0=0  reg_desc1=0  reg_desc2=0  reg_desc3=0  reg_desc4=0  reg_desc5=0  reg_desc6=0  reg_desc7=0  reg_addr=34  SampleTime=DSPBASampleTime  version=20090407
  dTheta_dt_Output : DSPBAModelBus/RegOut  reg_name=dTheta_dt  reg_rwmode=Read  reg_msb=wordLength - 1  reg_lsb=0  reg_desc=dTheta_dt rad_s output value  reg_addr=54  SampleTime=-1  version=20090407
  ia_Output : DSPBAModelBus/RegOut  reg_name=ia  reg_rwmode=Read  reg_msb=wordLength - 1  reg_lsb=0  reg_desc=ia output value  reg_addr=48  SampleTime=-1  version=20090407
  ib_Output : DSPBAModelBus/RegOut  reg_name=ib  reg_rwmode=Read  reg_msb=wordLength - 1  reg_lsb=0  reg_desc=ib output value  reg_addr=49  SampleTime=-1  version=20090407
  ic_Output : DSPBAModelBus/RegOut  reg_name=ic  reg_rwmode=Read  reg_msb=wordLength - 1  reg_lsb=0  reg_desc=ic output value  reg_addr=50  SampleTime=-1  version=20090407
  inv_J_CFG : DSPBAModelBus/RegField  reg_name=inv_J_cfg  reg_rwmode=Read/Write  reg_msb=wordLength - 1  reg_lsb=0  reg_mode=Specify via dialog  reg_type=ufix(16)  reg_scale=1  reg_init=0  reg_desc=inv_J_cfg input value  reg_modal=off  reg_desc0=0  reg_desc1=0  reg_desc2=0  reg_desc3=0  reg_desc4=0  reg_desc5=0  reg_desc6=0  reg_desc7=0  reg_addr=22  SampleTime=DSPBASampleTime  version=20090407
  inv_Lphase_CFG : DSPBAModelBus/RegField  reg_name=inv_Lphase_cfg  reg_rwmode=Read/Write  reg_msb=wordLength - 1  reg_lsb=0  reg_mode=Specify via dialog  reg_type=ufix(16)  reg_scale=2^-6  reg_init=0  reg_desc=inv_Lphase_cfg input value  reg_modal=off  reg_desc0=0  reg_desc1=0  reg_desc2=0  reg_desc3=0  reg_desc4=0  reg_desc5=0  reg_desc6=0  reg_desc7=0  reg_addr=18  SampleTime=DSPBASampleTime  version=20090407
  MM_valid_in : Outport
  Vabc_range_V_cfg : Outport  Port=2
  Va_V : Outport  Port=3
  Vb_V : Outport  Port=4
  Vc_V : Outport  Port=5
  SampleTime_s_cfg : Outport  Port=6
  Rphase_ohm_cfg : Outport  Port=7
  inv_Lphase_1_H_cfg : Outport  Port=8
  PolePairs_int_cfg : Outport  Port=9
  Ke_Vs_rad_cfg : Outport  Port=10
  Kt_Nm_A_cfg : Outport  Port=11
  inv_J_1_kgm2_cfg : Outport  Port=12
  LoadT_Nm : Outport  Port=13
  DC_link_range_V_cfg : Outport  Port=14
  DC_link_V : Outport  Port=15
  Iabc_range_cfg : Outport  Port=16
  wires:
  DSPBA_Start/1 -> Display1/1, GPOut/1
  GPOut/1 -> MM_valid_in/1
  GPOut1/1 -> SampleTime_s_cfg/1
  Sample_Time_CFG/1 -> Display/1, GPOut1/1
  GPOut2/1 -> Rphase_ohm_cfg/1
  Rphase_CFG/1 -> GPOut2/1
  GPOut3/1 -> inv_Lphase_1_H_cfg/1
  inv_Lphase_CFG/1 -> GPOut3/1
  PolePairs_CFG/1 -> GPOut4/1
  GPOut4/1 -> PolePairs_int_cfg/1
  Ke_CFG/1 -> GPOut5/1
  GPOut5/1 -> Ke_Vs_rad_cfg/1
  Kt_CFG/1 -> GPOut6/1
  GPOut6/1 -> Kt_Nm_A_cfg/1
  inv_J_CFG/1 -> GPOut7/1
  GPOut7/1 -> inv_J_1_kgm2_cfg/1
  GPOut8/1 -> Va_V/1
  Va_Input/1 -> GPOut8/1
  Vb_Input/1 -> GPOut9/1
  Vc_Input/1 -> GPOut10/1
  GPOut9/1 -> Vb_V/1
  GPOut10/1 -> Vc_V/1
  LoadT_Input/1 -> GPOut11/1
  GPOut11/1 -> LoadT_Nm/1
  DC_link_V_Input/1 -> GPOut12/1
  GPOut12/1 -> DC_link_V/1
  MM_valid_out/1 -> GPIn/1
  GPIn/1 -> DSPBA_Ready/2, ia_Output/2, ib_Output/2, ThetaMech_Output/2, dTheta_dt_Output/2, ic_Output/2, DSPBA_Ready/1
  ia_A/1 -> GPIn1/1
  GPIn1/1 -> ia_Output/1
  ib_A/1 -> GPIn2/1
  GPIn2/1 -> ib_Output/1
  ic_A/1 -> GPIn3/1
  GPIn3/1 -> ic_Output/1
  dTheta_dt_rad_s/1 -> GPIn4/1
  GPIn4/1 -> dTheta_dt_Output/1
  ThetaMech_one_turn/1 -> GPIn5/1
  GPIn5/1 -> ThetaMech_Output/1
  Constantdc2/1 -> DSPBA_Busy/2
  Not1/1 -> DSPBA_Busy/1
  ready/1 -> GPIn6/1
  GPIn6/1 -> Not1/1
  GPOut13/1 -> Vabc_range_V_cfg/1
  Vabc_range_CFG/1 -> GPOut13/1
  GPOut14/1 -> DC_link_range_V_cfg/1
  DC_link_range_CFG/1 -> GPOut14/1
  GPOut15/1 -> Iabc_range_cfg/1
  Iabc_range_CFG/1 -> GPOut15/1

== system motor_kit_sim_20MHz/MotorModel/Current_scale_64_ ==
  note: Motor phase currents 16 bits Sigma-Delta ADC (ADC interface:16 bits . Interface rtl: ip\ssg_emb_sd_adc ) : 1024 counts/A. Data type:sfix16_En10. Convert this value to range 0 to 1 (ufix16_En16). 2^16/1024 = 64; 2^15/1024 = 32. This means -32A will be 0 and 32A will be 1.
      | Schematic page 12: +/-32A current measurement. Current is sensed across 0.01 resistor. I=V/R = V/0.01 = 100*V
      | Motor phase currents Intel MAX10 ADC: 81.9 counts/A, convert this value to 16 bits, same as Sigma-Delta ADC:
      | MAX10 ADC read back value * 1024/81.9 = MAX10 ADC read back value * 12803/1024
  Current_range_int16 : Inport
  Current_sfix16_En10 : Inport  Port=2
  Add1 : DSPBAPrim/Add  primtype=add  nInputs=evalAionMaskParam(gcb,'value',1)  nOutputs=1  omode=Inherit via internal rule with word growth  otype=sfix(16)  scale=2^-15  rndmethod=Unbiased  factor=1  satmethod=Symmetric  shift_vec=[0 1 2 -1]  value=2  inPortNames=[' '; ' ';]  outPortNames=[' ']  dspbaimage=dspba_prim.svg  text=fprintf('+');  style=Optimised  visibilities=1032+2^17+2^18+2^19  genFPC=off  floatRounding=correct  advOptions=[]  version=20211007
  Const1 : DSPBAPrim/Const  primtype=const  nInputs=0  nOutputs=1  omode=Specify via dialog  otype=DataType  scale=constScaleFraction  rndmethod=Unbiased  factor=1  satmethod=Symmetric  shift_vec=[0 1 2 -1]  value=1/2  inPortNames=['+'; '+';]  outPortNames=[' ']  dspbaimage=dspba_prim.svg  text=fprintf('%s', num2str(value));  style=Optimised  visibilities=8 + 1024  floatPrecision=float32_m23  warnSaturation=on  version=20211007  SampleTime=inf
  Convert4 : DSPBAPrim/Convert  primtype=convert  nInputs=1  nOutputs=1  omode=Specify via dialog  otype=DataTypeFraction  scale=constScaleFraction  rndmethod=Biased  factor=1  satmethod=None  shift_vec=[0 1 2 -1]  value=round([0:255]/17)  inPortNames=[' '; ' ';]  outPortNames=[' '; 'c']  dspbaimage=dspba_prim_wide.svg  text=fprintf('convert');  style=Optimised  visibilities=8+64+256+2^17  clipdetect=off  floatPrecision=float32_m23  advOptions=[]  version=20211007
  Divide : DSPBAPrim/Divide  primtype=divide  nInputs=2  nOutputs=1  omode=Inherit via internal rule  otype=sfix(16)  scale=2^-15  rndmethod=Unbiased  factor=1  satmethod=Symmetric  shift_vec=[0 1 2 -1]  value=round([0:255]/17)  inPortNames=[' '; ' ';]  outPortNames=[' ']  dspbaimage=dspba_prim.svg  text=fprintf('a\n----\nb');  style=Optimised  visibilities=8+2^17+2^18  floatRounding=correct  intDivider=off  advOptions=[]  version=20211007
  GPIn : DSPBAPrim/GPIn  primtype=gpin  nInputs=evalAionMaskParam(gcb,'value',1)  nOutputs=evalAionMaskParam(gcb,'value',1)  omode=Inherit via internal rule  otype=sfix(16)  scale=2^-15  rndmethod=Unbiased  factor=1  satmethod=Symmetric  shift_vec=[0 1 2 -1]  value=1  inPortNames=[' ' ' ' ' ' ' ' ' ' ' ' ' ' ' ' ' ' ' ' ' ' ' ' ' ' ' ' ' ' ' ' ' ' ' ' ' ' ' ' ' ' ' ' ' ' ' ' ' ' ' ' ' ' ' ' ' ' ' ' ' ' ' ' ' ' ' ' ' ']'  outPortNames=[' ' ' ' ' ' ' ' ' ' ' ' ' ' ' ' ' ' ' ' ' ' ' ' ' ' ' ' ' ' ' ' ' ' ' ' ' ' ' ' ' ' ' ' ' ' ' ' ' ' ' ' ' ' ' ' ' ' ' ' ' ' ' ' ' ' ' ' ' ']'  dspbaimage=dspba_prim_channel_tall.svg  text=fprintf('GPIn');  style=Optimised  visibilities=1024  scheduleOrigin=off  version=20211214
  GPIn1 : DSPBAPrim/GPIn  primtype=gpin  nInputs=evalAionMaskParam(gcb,'value',1)  nOutputs=evalAionMaskParam(gcb,'value',1)  omode=Inherit via internal rule  otype=sfix(16)  scale=2^-15  rndmethod=Unbiased  factor=1  satmethod=Symmetric  shift_vec=[0 1 2 -1]  value=1  inPortNames=[' ' ' ' ' ' ' ' ' ' ' ' ' ' ' ' ' ' ' ' ' ' ' ' ' ' ' ' ' ' ' ' ' ' ' ' ' ' ' ' ' ' ' ' ' ' ' ' ' ' ' ' ' ' ' ' ' ' ' ' ' ' ' ' ' ' ' ' ' ']'  outPortNames=[' ' ' ' ' ' ' ' ' ' ' ' ' ' ' ' ' ' ' ' ' ' ' ' ' ' ' ' ' ' ' ' ' ' ' ' ' ' ' ' ' ' ' ' ' ' ' ' ' ' ' ' ' ' ' ' ' ' ' ' ' ' ' ' ' ' ' ' ' ']'  dspbaimage=dspba_prim_channel_tall.svg  text=fprintf('GPIn');  style=Optimised  visibilities=1024  scheduleOrigin=off  version=20211214
  GPOut : DSPBAPrim/GPOut  primtype=gpout  nInputs=evalAionMaskParam(gcb,'value',1)  nOutputs=evalAionMaskParam(gcb,'value',1)  omode=Inherit via internal rule  otype=sfix(16)  scale=2^-15  rndmethod=Unbiased  factor=1  satmethod=Symmetric  shift_vec=[0 1 2 -1]  value=1  inPortNames=[' ' ' ' ' ' ' ' ' ' ' ' ' ' ' ' ' ' ' ' ' ' ' ' ' ' ' ' ' ' ' ' ' ' ' ' ' ' ' ' ' ' ' ' ' ' ' ' ' ' ' ' ' ' ' ' ' ' ' ' ' ' ' ' ' ' ' ' ' ']'  outPortNames=[' ' ' ' ' ' ' ' ' ' ' ' ' ' ' ' ' ' ' ' ' ' ' ' ' ' ' ' ' ' ' ' ' ' ' ' ' ' ' ' ' ' ' ' ' ' ' ' ' ' ' ' ' ' ' ' ' ' ' ' ' ' ' ' ' ' ' ' ' ']'  dspbaimage=dspba_prim_channel_tall.svg  text=fprintf('GPOut');  style=Optimised  visibilities=1024  latency=13  version=20211214
  Mult : DSPBAPrim/Mult  primtype=mult  nInputs=2  nOutputs=1  omode=Inherit via internal rule  otype=sfix(16)  scale=2^-15  rndmethod=Unbiased  factor=1  satmethod=Symmetric  shift_vec=[0 1 2 -1]  value=0  inPortNames=[' '; ' ';]  outPortNames=[' ']  dspbaimage=dspba_prim.svg  text=fprintf('X');  style=Optimised  visibilities=8+2^18+2^19  floatPrecision=float32_m23  floatRounding=correct  advOptions=[]  version=20211007
  SynthesisInfo1 : DSPBAPrim/SynthesisInfo  primtype=synthinfo  nInputs=0  nOutputs=0  omode=Inherit via internal rule  otype=sfix(16)  scale=2^-15  rndmethod=Truncate  factor=1  satmethod=Symmetric  shift_vec=[0 1 2 -1]  value=99  inPortNames=[' '; ' ';]  outPortNames=[' ']  dspbaimage=dspba_prim_ctrl.jpg  text=fprintf('Style=%s', style);  style=Scheduled  visibilities=2^17+2^18+2^19+2^20  constraintPair=None  constraintRelation=>  constraintLimit=2  modelRefSign=+  modelRef=''  showSchedule=off  simulationMode=Use Global Value  resetMinimization=Conditional - On for ChannelIn/Out only  version=20220106
  "Fraction_ND_ufix16_En16 " : Outport
  wires:
  Mult/1 -> Convert4/1
  GPIn1/1 -> Add1/2
  Divide/1 -> Mult/1
  Current_range_int16/1 -> GPIn/1
  Add1/1 -> Mult/2
  Convert4/1 -> GPOut/1
  GPOut/1 -> "Fraction_ND_ufix16_En16 "/1
  GPIn/1 -> Divide/2, Add1/1
  Const1/1 -> Divide/1
  Current_sfix16_En10/1 -> GPIn1/1

== system motor_kit_sim_20MHz/MotorModel/Current_scale_64_1 ==
  note: Motor phase currents 16 bits Sigma-Delta ADC (ADC interface:16 bits . Interface rtl: ip\ssg_emb_sd_adc ) : 1024 counts/A. Data type:sfix16_En10. Convert this value to range 0 to 1 (ufix16_En16). 2^16/1024 = 64; 2^15/1024 = 32. This means -32A will be 0 and 32A will be 1.
      | Schematic page 12: +/-32A current measurement. Current is sensed across 0.01 resistor. I=V/R = V/0.01 = 100*V
      | Motor phase currents Intel MAX10 ADC: 81.9 counts/A, convert this value to 16 bits, same as Sigma-Delta ADC:
      | MAX10 ADC read back value * 1024/81.9 = MAX10 ADC read back value * 12803/1024
  Current_range_int16 : Inport
  Current_sfix16_En10 : Inport  Port=2
  Add1 : DSPBAPrim/Add  primtype=add  nInputs=evalAionMaskParam(gcb,'value',1)  nOutputs=1  omode=Inherit via internal rule with word growth  otype=sfix(16)  scale=2^-15  rndmethod=Unbiased  factor=1  satmethod=Symmetric  shift_vec=[0 1 2 -1]  value=2  inPortNames=[' '; ' ';]  outPortNames=[' ']  dspbaimage=dspba_prim.svg  text=fprintf('+');  style=Optimised  visibilities=1032+2^17+2^18+2^19  genFPC=off  floatRounding=correct  advOptions=[]  version=20211007
  Const1 : DSPBAPrim/Const  primtype=const  nInputs=0  nOutputs=1  omode=Specify via dialog  otype=DataType  scale=constScaleFraction  rndmethod=Unbiased  factor=1  satmethod=Symmetric  shift_vec=[0 1 2 -1]  value=1/2  inPortNames=['+'; '+';]  outPortNames=[' ']  dspbaimage=dspba_prim.svg  text=fprintf('%s', num2str(value));  style=Optimised  visibilities=8 + 1024  floatPrecision=float32_m23  warnSaturation=on  version=20211007  SampleTime=inf
  Convert4 : DSPBAPrim/Convert  primtype=convert  nInputs=1  nOutputs=1  omode=Specify via dialog  otype=DataTypeFraction  scale=constScaleFraction  rndmethod=Biased  factor=1  satmethod=None  shift_vec=[0 1 2 -1]  value=round([0:255]/17)  inPortNames=[' '; ' ';]  outPortNames=[' '; 'c']  dspbaimage=dspba_prim_wide.svg  text=fprintf('convert');  style=Optimised  visibilities=8+64+256+2^17  clipdetect=off  floatPrecision=float32_m23  advOptions=[]  version=20211007
  Divide : DSPBAPrim/Divide  primtype=divide  nInputs=2  nOutputs=1  omode=Inherit via internal rule  otype=sfix(16)  scale=2^-15  rndmethod=Unbiased  factor=1  satmethod=Symmetric  shift_vec=[0 1 2 -1]  value=round([0:255]/17)  inPortNames=[' '; ' ';]  outPortNames=[' ']  dspbaimage=dspba_prim.svg  text=fprintf('a\n----\nb');  style=Optimised  visibilities=8+2^17+2^18  floatRounding=correct  intDivider=off  advOptions=[]  version=20211007
  GPIn : DSPBAPrim/GPIn  primtype=gpin  nInputs=evalAionMaskParam(gcb,'value',1)  nOutputs=evalAionMaskParam(gcb,'value',1)  omode=Inherit via internal rule  otype=sfix(16)  scale=2^-15  rndmethod=Unbiased  factor=1  satmethod=Symmetric  shift_vec=[0 1 2 -1]  value=1  inPortNames=[' ' ' ' ' ' ' ' ' ' ' ' ' ' ' ' ' ' ' ' ' ' ' ' ' ' ' ' ' ' ' ' ' ' ' ' ' ' ' ' ' ' ' ' ' ' ' ' ' ' ' ' ' ' ' ' ' ' ' ' ' ' ' ' ' ' ' ' ' ']'  outPortNames=[' ' ' ' ' ' ' ' ' ' ' ' ' ' ' ' ' ' ' ' ' ' ' ' ' ' ' ' ' ' ' ' ' ' ' ' ' ' ' ' ' ' ' ' ' ' ' ' ' ' ' ' ' ' ' ' ' ' ' ' ' ' ' ' ' ' ' ' ' ']'  dspbaimage=dspba_prim_channel_tall.svg  text=fprintf('GPIn');  style=Optimised  visibilities=1024  scheduleOrigin=off  version=20211214
  GPIn1 : DSPBAPrim/GPIn  primtype=gpin  nInputs=evalAionMaskParam(gcb,'value',1)  nOutputs=evalAionMaskParam(gcb,'value',1)  omode=Inherit via internal rule  otype=sfix(16)  scale=2^-15  rndmethod=Unbiased  factor=1  satmethod=Symmetric  shift_vec=[0 1 2 -1]  value=1  inPortNames=[' ' ' ' ' ' ' ' ' ' ' ' ' ' ' ' ' ' ' ' ' ' ' ' ' ' ' ' ' ' ' ' ' ' ' ' ' ' ' ' ' ' ' ' ' ' ' ' ' ' ' ' ' ' ' ' ' ' ' ' ' ' ' ' ' ' ' ' ' ']'  outPortNames=[' ' ' ' ' ' ' ' ' ' ' ' ' ' ' ' ' ' ' ' ' ' ' ' ' ' ' ' ' ' ' ' ' ' ' ' ' ' ' ' ' ' ' ' ' ' ' ' ' ' ' ' ' ' ' ' ' ' ' ' ' ' ' ' ' ' ' ' ' ']'  dspbaimage=dspba_prim_channel_tall.svg  text=fprintf('GPIn');  style=Optimised  visibilities=1024  scheduleOrigin=off  version=20211214
  GPOut : DSPBAPrim/GPOut  primtype=gpout  nInputs=evalAionMaskParam(gcb,'value',1)  nOutputs=evalAionMaskParam(gcb,'value',1)  omode=Inherit via internal rule  otype=sfix(16)  scale=2^-15  rndmethod=Unbiased  factor=1  satmethod=Symmetric  shift_vec=[0 1 2 -1]  value=1  inPortNames=[' ' ' ' ' ' ' ' ' ' ' ' ' ' ' ' ' ' ' ' ' ' ' ' ' ' ' ' ' ' ' ' ' ' ' ' ' ' ' ' ' ' ' ' ' ' ' ' ' ' ' ' ' ' ' ' ' ' ' ' ' ' ' ' ' ' ' ' ' ']'  outPortNames=[' ' ' ' ' ' ' ' ' ' ' ' ' ' ' ' ' ' ' ' ' ' ' ' ' ' ' ' ' ' ' ' ' ' ' ' ' ' ' ' ' ' ' ' ' ' ' ' ' ' ' ' ' ' ' ' ' ' ' ' ' ' ' ' ' ' ' ' ' ']'  dspbaimage=dspba_prim_channel_tall.svg  text=fprintf('GPOut');  style=Optimised  visibilities=1024  latency=13  version=20211214
  Mult : DSPBAPrim/Mult  primtype=mult  nInputs=2  nOutputs=1  omode=Inherit via internal rule  otype=sfix(16)  scale=2^-15  rndmethod=Unbiased  factor=1  satmethod=Symmetric  shift_vec=[0 1 2 -1]  value=0  inPortNames=[' '; ' ';]  outPortNames=[' ']  dspbaimage=dspba_prim.svg  text=fprintf('X');  style=Optimised  visibilities=8+2^18+2^19  floatPrecision=float32_m23  floatRounding=correct  advOptions=[]  version=20211007
  SynthesisInfo1 : DSPBAPrim/SynthesisInfo  primtype=synthinfo  nInputs=0  nOutputs=0  omode=Inherit via internal rule  otype=sfix(16)  scale=2^-15  rndmethod=Truncate  factor=1  satmethod=Symmetric  shift_vec=[0 1 2 -1]  value=99  inPortNames=[' '; ' ';]  outPortNames=[' ']  dspbaimage=dspba_prim_ctrl.jpg  text=fprintf('Style=%s', style);  style=Scheduled  visibilities=2^17+2^18+2^19+2^20  constraintPair=None  constraintRelation=>  constraintLimit=2  modelRefSign=+  modelRef=''  showSchedule=off  simulationMode=Use Global Value  resetMinimization=Conditional - On for ChannelIn/Out only  version=20220106
  "Fraction_ND_ufix16_En16 " : Outport
  wires:
  Mult/1 -> Convert4/1
  GPIn1/1 -> Add1/2
  Divide/1 -> Mult/1
  Current_range_int16/1 -> GPIn/1
  Add1/1 -> Mult/2
  Convert4/1 -> GPOut/1
  GPOut/1 -> "Fraction_ND_ufix16_En16 "/1
  GPIn/1 -> Divide/2, Add1/1
  Const1/1 -> Divide/1
  Current_sfix16_En10/1 -> GPIn1/1
